simulink model "Torque_Vectoring_Controller_Boon"  (R2016a)
settings: Solver=ode45  StartTime=0.0  StopTime=inf  RelTol=1e-3
InitFcn:
  | clear_close
  | dataCar
  | optParam
  | structSensors
  | structSettings
  | structEstimPar
  | structAero
  | structVariables
  | readFuzzyFile
StartFcn:
  | clear_close
  | dataCar
  | optParam
  | structSensors
  | structSettings
  | structEstimPar
  | structAero
  | structVariables
  | readFuzzyFile
values from neighbouring files (symbols this model uses):
  mu = [0.05;0.05;0.05;0.05]    [frictionfrank.m]
undefined symbols (not defined in the file or in its folder): car, optPar, tire_radius
libraries: CarMaker4SL x42, simulink x11, fuzblock x1
(part 1 of 3)
settings Model: ExtModeAutoUpdateStatusClock=off  Creator=fh  LastModifiedBy=Boon
settings DataIOCC: LimitDataPoints=on  SaveFormat=Array  SignalLoggingSaveFormat=ModelDataLogs  SignalLoggingName=sigsOut
settings OptimizationCC: BooleanDataType=off  ExpressionDepthLimit=2147483647  InitFltsAndDblsToZero=on
settings DebuggingCC: SaveWithParameterizedLinksMsg=none  UnderspecifiedInitializationDetection=Classic  MergeDetectMultiDrivingBlocksExec=none  SignalResolutionControl=TryResolveAllWithWarning  MultiTaskDSMMsg=warning  MultiTaskCondExecSysMsg=none  FcnCallInpInsideContextMsg=EnableAllAsWarning  StateNameClashWarn=warning
settings HardwareCC: ProdBitPerPointer=32  ProdLargestAtomicFloat=None  ProdIntDivRoundTo=Undefined  ProdEndianess=Unspecified  ProdWordSize=32  ProdHWDeviceType=32-bit Generic  TargetUnknown=on
settings ModelReferenceCC: PropagateSignalLabelsOutOfModel=off
settings CodeAppCC: MaxIdLength=63
settings GRTTargetCC: TargetFcnLib=ansi_tfl_tmw.mat  CombineOutputUpdateFcns=off  GRTInterface=on

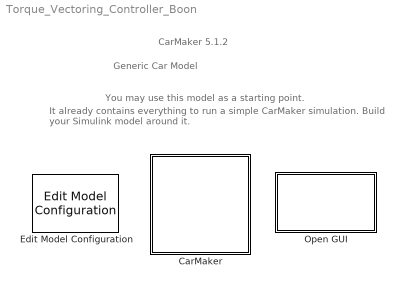
== system Torque_Vectoring_Controller_Boon ==
  note: Generic Car Model
  note: You may use this model as a starting point.
  note: It already contains everything to run a simple CarMaker simulation.
      | Build your Simulink model around it.
  note: CarMaker 5.1.2
  CarMaker : Subsystem  TreatAsAtomicUnit=on
      mask Display: image(imread('CarMaker4SLss.bmp'));
  Edit Model Configuration : CarMaker4SL/Edit Model Configuration
  Open GUI : Subsystem  LoadFcn=if ~length(which('cmcmd')), cmenv; end
      settings: OpenFcn=cmblockmagic('gui_fix_display'); CM_Simulink
      mask Display: image(imread('CarMakerGUI.bmp'));

== system Torque_Vectoring_Controller_Boon/CarMaker ==
  CM_FIRST : Subsystem
  CM_LAST : Subsystem
  Controls : Subsystem
  DrivMan : Subsystem
  Ground : Ground
  IPG Feedback : Subsystem
  IPG Vehicle : Subsystem  TreatAsAtomicUnit=on
  Terminator : Terminator
  Vehicle Sensors : Subsystem
  VehicleControl : Subsystem
  Write CM Dict : CarMaker4SL/Write CM Dict  Commented=on  xname=PT.WFL.Trq_Drive  xsync=off
  Write CM Dict1 : CarMaker4SL/Write CM Dict  Commented=on  xname=PT.WFR.Trq_Drive  xsync=off
  Write CM Dict2 : CarMaker4SL/Write CM Dict  Commented=on  xname=PT.WRL.Trq_Drive  xsync=off
  Write CM Dict3 : CarMaker4SL/Write CM Dict  Commented=on  xname=PT.WRR.Trq_Drive  xsync=off
  wires:
  DrivMan/2(DrivMan.Out) -> VehicleControl/2(DrivMan.In)
  DrivMan/1(Sync_Out) -> VehicleControl/1(Sync_In)
  CM_FIRST/2(Env.Misc) -> DrivMan/2(Env.Misc)
  CM_FIRST/1(Sync_Out) -> DrivMan/1(Sync_In)
  CM_LAST/1(Sync_Out) -> Terminator/1
  IPG Vehicle/1(Sync_Out) -> CM_LAST/1(Sync_In)
  VehicleControl/1(Sync_Out) -> IPG Vehicle/1(Sync_In)
  VehicleControl/3(VhclCtrl.Steering) -> IPG Vehicle/3(VhclCtrl.Steering)
  VehicleControl/4(Vhcl.Wheel.In) -> IPG Vehicle/4(Vhcl.Wheel.In)
  VehicleControl/5(Vhcl.Misc) -> IPG Vehicle/5(Vhcl.Misc)
  VehicleControl/6(VhclCtrl.Brake) -> IPG Vehicle/6(VhclCtrl.Brake)
  VehicleControl/7(VhclCtrl.PT) -> IPG Vehicle/7(VhclCtrl.PT)
  VehicleControl/2(Vhcl.Model.Source) -> IPG Vehicle/2(Vhcl.Model.Source)
  Ground/1 -> CM_FIRST/1(Sync_In)
  Vehicle Sensors/1(" Sensor Bus") -> Controls/1(Sensor Bus)
  Controls/1(Torque Bus) -> IPG Feedback/1(Torques)
  Vehicle Sensors/2(wheelspeeds) -> IPG Feedback/2(Wheelspeeds)

== system Torque_Vectoring_Controller_Boon/Open GUI ==
  S-Function : S-Function  FunctionName=cm_gui  SFunctionDeploymentMode=off  EnableBusSupport=off

== system Torque_Vectoring_Controller_Boon/CarMaker/CM_FIRST ==
  Sync_In : Inport
  Bus Creator1 : BusCreator  Inputs=9
  Demux : Demux  Outputs=9
  Environment : S-Function  FunctionName=CM_Sfun  Parameters='Environment'  SFunctionDeploymentMode=off  EnableBusSupport=off
  IoIn : S-Function  FunctionName=CM_Sfun  Parameters='IoIn'  SFunctionDeploymentMode=off  EnableBusSupport=off
  Sync_Out : Outport
  Env.Misc : Outport  Port=2
  wires:
  Bus Creator1/1 -> Env.Misc/1
  Environment/2 -> Demux/1
  Demux/4 -> Bus Creator1/4  "Env AirHumidity"
  Demux/3 -> Bus Creator1/3  "Env AirPressure"
  Demux/2 -> Bus Creator1/2  "Env AirDensity"
  Demux/1 -> Bus Creator1/1  "Env Temperature"
  Environment/1 -> Sync_Out/1
  IoIn/1 -> Environment/1
  Sync_In/1 -> IoIn/1
  Demux/5 -> Bus Creator1/5  "Env Time"
  Demux/6 -> Bus Creator1/6  "Env SolarRadiation"
  Demux/7 -> Bus Creator1/7  "Env WindVel_tot x"
  Demux/8 -> Bus Creator1/8  "Env WindVel_tot y"
  Demux/9 -> Bus Creator1/9  "Env WindVel_tot z"

== system Torque_Vectoring_Controller_Boon/CarMaker/CM_LAST ==
  Sync_In : Inport
  CM_User : S-Function  FunctionName=CM_Sfun  Parameters='CM_User'  SFunctionDeploymentMode=off  EnableBusSupport=off
  IoOut : S-Function  FunctionName=CM_Sfun  Parameters='IoOut'  SFunctionDeploymentMode=off  EnableBusSupport=off
  Sync_Out : Outport
  wires:
  IoOut/1 -> Sync_Out/1
  CM_User/1 -> IoOut/1
  Sync_In/1 -> CM_User/1

== system Torque_Vectoring_Controller_Boon/CarMaker/Controls ==
  Sensor Bus : Inport
  Control Systems : Subsystem
  Controller Settings : Subsystem
  Vehicle Estimated Parameters : Subsystem
  Torque Bus : Outport
  wires:
  Control Systems/1(Torques) -> Torque Bus/1
  Sensor Bus/1 -> Controller Settings/1(Sensor Bus), Control Systems/1(Sensor Bus), Vehicle Estimated Parameters/1(Sensor Bus)
  [Settings] -> Vehicle Estimated Parameters/2(Settings)
  Vehicle Estimated Parameters/1(" estimParBus") -> Control Systems/4(estimParBus)
  Controller Settings/1(Settings) -> [Settings]
  [Settings] -> Control Systems/2(Settings)
  Controller Settings/2(Variables) -> [Variables]
  [Variables] -> Control Systems/3("Variables ")

== system Torque_Vectoring_Controller_Boon/CarMaker/DrivMan ==
  note: There's rarely a reason to override DrivMan signals.
      | Use the VehicleControl interface for this purpose.
  Sync_In : Inport
  Env.Misc : Inport  Port=2
  BusCreator : BusCreator  Inputs=17
  Demux : Demux  Outputs=17
  DrivMan : S-Function  FunctionName=CM_Sfun  Parameters='DrivMan'  SFunctionDeploymentMode=off  EnableBusSupport=off
  Sync_Out : Outport
  DrivMan.Out : Outport  Port=2
  wires:
  Demux/17 -> BusCreator/17  "DrivMan Steering Trq"
  Demux/16 -> BusCreator/16  "DrivMan Steering AngAcc"
  Demux/15 -> BusCreator/15  "DrivMan Steering AngVel"
  Demux/14 -> BusCreator/14  "DrivMan Steering Ang"
  Demux/13 -> BusCreator/13  "DrivMan Gas"
  Demux/12 -> BusCreator/12  "DrivMan Clutch"
  Demux/11 -> BusCreator/11  "DrivMan BrakePark"
  Demux/10 -> BusCreator/10  "DrivMan Brake"
  Demux/9 -> BusCreator/9  "DrivMan GearNo"
  Demux/8 -> BusCreator/8  "DrivMan SelectorCtrl"
  Demux/7 -> BusCreator/7  "DrivMan UserSignal4"
  Demux/6 -> BusCreator/6  "DrivMan UserSignal3"
  Demux/5 -> BusCreator/5  "DrivMan UserSignal2"
  Demux/4 -> BusCreator/4  "DrivMan UserSignal1"
  Demux/3 -> BusCreator/3  "DrivMan UserSignal0"
  Demux/2 -> BusCreator/2  "DrivMan Key"
  Demux/1 -> BusCreator/1  "DrivMan SST"
  Env.Misc/1 -> DrivMan/2
  Sync_In/1 -> DrivMan/1
  DrivMan/1 -> Sync_Out/1
  BusCreator/1 -> DrivMan.Out/1
  DrivMan/2 -> Demux/1

== system Torque_Vectoring_Controller_Boon/CarMaker/IPG Feedback ==
  Torques : Inport
  Wheelspeeds : Inport  Port=2
  Constant : Constant  Value=1200  VectorParams1D=off  SampleTime=-1
  Demux : Demux
  Subsystem : Subsystem
  wires:
  Demux/3 -> Subsystem/3(Torque_MotRL)
  Torques/1 -> Demux/1
  Constant/1 -> Subsystem/8(WheelspeedLimitRR_RPM), Subsystem/7(WheelspeedLimitRL_RPM), Subsystem/6(WheelspeedLimitFR_RPM), Subsystem/5(WheelspeedLimitFL_RPM)
  Demux/2 -> Subsystem/2(Torque_MotFR)
  Wheelspeeds/1 -> Subsystem/9(SensorBus)
  Demux/1 -> Subsystem/1(Torque_MotFL)
  Demux/4 -> Subsystem/4(Torque_MotRR)

== system Torque_Vectoring_Controller_Boon/CarMaker/IPG Vehicle ==
  Sync_In : Inport
  Vhcl.Model.Source : Inport  Port=2
  VhclCtrl.Steering : Inport  Port=3
  Vhcl.Wheel.In : Inport  Port=4
  Vhcl.Misc : Inport  Port=5
  VhclCtrl.Brake : Inport  Port=6
  VhclCtrl.PT : Inport  Port=7
  Brake : Subsystem
  CarAndTrailer : Subsystem
  PowerTrain : Subsystem
  Stop Simulation : Stop
  VehicleSource_BuiltIn : simulink/Logic and Bit Operations/Compare To Constant  relop=~=  const=1  OutDataTypeStr=boolean  ZeroCross=off
  Sync_Out : Outport
  wires:
  VhclCtrl.PT/1 -> PowerTrain/3(VhclCtrl.PT)
  Brake/1(Sync_Out) -> PowerTrain/1(Sync_In)
  CarAndTrailer/1(Sync_Out) -> Brake/1(Sync_In)
  CarAndTrailer/2(Brake.IF.In) -> Brake/2(Brake.IF.In)
  VhclCtrl.Brake/1 -> Brake/3(VhclCtrl.Brake)
  PowerTrain/1(Sync_Out) -> Sync_Out/1
  Vhcl.Misc/1 -> CarAndTrailer/4(Vhcl.Misc)
  Vhcl.Wheel.In/1 -> CarAndTrailer/3(Vhcl.Wheel.In)
  VhclCtrl.Steering/1 -> CarAndTrailer/2(VhclCtrl.Steering)
  Sync_In/1 -> CarAndTrailer/1(Sync_In)
  Vhcl.Model.Source/1 -> VehicleSource_BuiltIn/1
  VehicleSource_BuiltIn/1 -> Stop Simulation/1
  Brake/2(Vhcl.Wheel.PT) -> PowerTrain/2(Vhcl.Wheel.PT)

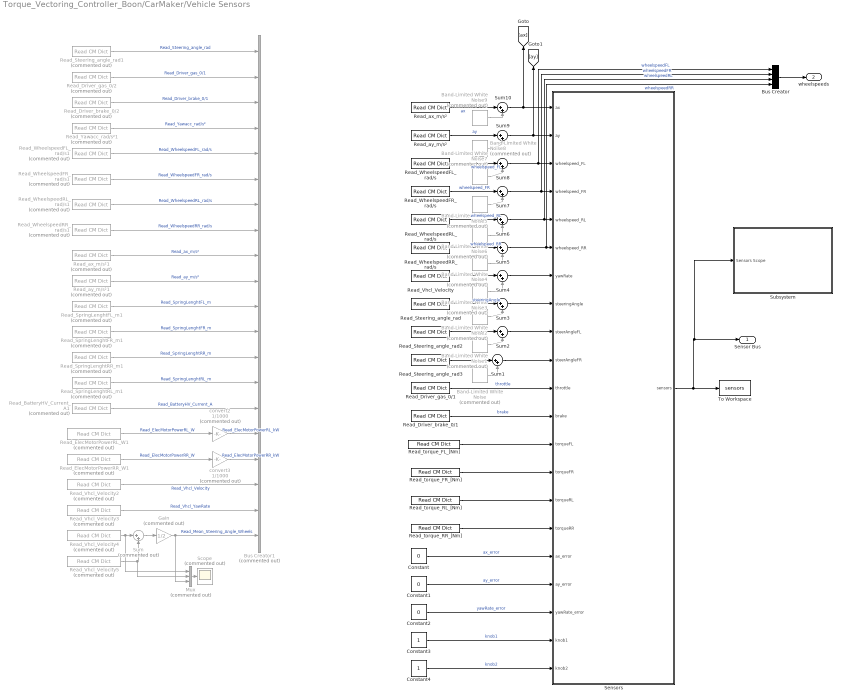
== system Torque_Vectoring_Controller_Boon/CarMaker/Vehicle Sensors ==
  Band-Limited White Noise{,1..9} (10 alike) : simulink/Sources/Band-Limited White Noise  Commented=on  Cov=[0.00000001]  Ts=car.dt  seed=[23341]
  Bus Creator : BusCreator  Inputs=4
  Bus Creator1 : BusCreator  Commented=on  Inputs=20
  Constant : Constant  Value=0
  Constant1 : Constant  Value=0
  Constant2 : Constant  Value=0
  Constant3 : Constant
  Constant4 : Constant
  Gain : Gain  Commented=on  Gain=1/2
  Mux : Mux  Commented=on  Inputs=3
  Read_BatteryHV_Current_A1 : CarMaker4SL/Read CM Dict  Commented=on  xname=PT.BattHV.Current  xsync=off
  Read_Driver_brake_0/1 : CarMaker4SL/Read CM Dict  xname=DM.Brake  xsync=off
  Read_Driver_brake_0/2 : CarMaker4SL/Read CM Dict  Commented=on  xname=DM.Brake  xsync=off
  Read_Driver_gas_0/1 : CarMaker4SL/Read CM Dict  xname=DM.Gas  xsync=off
  Read_Driver_gas_0/2 : CarMaker4SL/Read CM Dict  Commented=on  xname=DM.Gas  xsync=off
  Read_ElecMotorPowerRL_W1 : CarMaker4SL/Read CM Dict  Commented=on  xname=PT.Motor.PwrElec  xsync=off
  Read_ElecMotorPowerRR_W1 : CarMaker4SL/Read CM Dict  Commented=on  xname=PT.Motor1.PwrElec  xsync=off
  Read_SpringLenghtFL_m1 : CarMaker4SL/Read CM Dict  Commented=on  xname=Car.SpringFL.l  xsync=off
  Read_SpringLenghtFR_m1 : CarMaker4SL/Read CM Dict  Commented=on  xname=Car.SpringFR.l  xsync=off
  Read_SpringLenghtRL_m1 : CarMaker4SL/Read CM Dict  Commented=on  xname=Car.SpringRL.l  xsync=off
  Read_SpringLenghtRR_m1 : CarMaker4SL/Read CM Dict  Commented=on  xname=Car.SpringRR.l  xsync=off
  Read_Steering_angle_rad : CarMaker4SL/Read CM Dict  xname=Steer.WhlAng  xsync=off
  Read_Steering_angle_rad1 : CarMaker4SL/Read CM Dict  Commented=on  xname=Steer.WhlAng  xsync=off
  Read_Steering_angle_rad2 : CarMaker4SL/Read CM Dict  xname=Car.SteerAngleFL  xsync=off
  Read_Steering_angle_rad3 : CarMaker4SL/Read CM Dict  xname=Car.SteerAngleFR  xsync=off
  Read_Vhcl_Velocity : CarMaker4SL/Read CM Dict  xname=Vhcl.YawRate  xsync=off
  Read_Vhcl_Velocity2 : CarMaker4SL/Read CM Dict  Commented=on  xname=Vhcl.v  xsync=off
  Read_Vhcl_Velocity3 : CarMaker4SL/Read CM Dict  Commented=on  xname=Vhcl.YawRate  xsync=off
  Read_Vhcl_Velocity4 : CarMaker4SL/Read CM Dict  Commented=on  xname=Car.SteerAngleFL  xsync=off
  Read_Vhcl_Velocity5 : CarMaker4SL/Read CM Dict  Commented=on  xname=Car.SteerAngleFR  xsync=off
  Read_WheelspeedFL_rad/s : CarMaker4SL/Read CM Dict  xname=Vhcl.FL.rotv  xsync=off
  Read_WheelspeedFL_rad/s1 : CarMaker4SL/Read CM Dict  Commented=on  xname=Vhcl.FL.rotv  xsync=off
  Read_WheelspeedFR_rad/s : CarMaker4SL/Read CM Dict  xname=Vhcl.FR.rotv  xsync=off
  Read_WheelspeedFR_rad/s1 : CarMaker4SL/Read CM Dict  Commented=on  xname=Vhcl.FR.rotv  xsync=off
  Read_WheelspeedRL_rad/s : CarMaker4SL/Read CM Dict  xname=Vhcl.RL.rotv  xsync=off
  Read_WheelspeedRL_rad/s1 : CarMaker4SL/Read CM Dict  Commented=on  xname=Vhcl.RL.rotv  xsync=off
  Read_WheelspeedRR_rad/s : CarMaker4SL/Read CM Dict  xname=Vhcl.RR.rotv  xsync=off
  Read_WheelspeedRR_rad/s1 : CarMaker4SL/Read CM Dict  Commented=on  xname=Vhcl.RR.rotv  xsync=off
  Read_Yawacc_rad/s²1 : CarMaker4SL/Read CM Dict  Commented=on  xname=Vhcl.YawAcc  xsync=off
  Read_ax_m/s² : CarMaker4SL/Read CM Dict  xname=Car.ax  xsync=off
  Read_ax_m/s²1 : CarMaker4SL/Read CM Dict  Commented=on  xname=Car.ax  xsync=off
  Read_ay_m/s² : CarMaker4SL/Read CM Dict  xname=Car.ay  xsync=off
  Read_ay_m/s²1 : CarMaker4SL/Read CM Dict  Commented=on  xname=Car.ay  xsync=off
  Read_torque_FL_[Nm] : CarMaker4SL/Read CM Dict  xname=PT.WFL.Trq_Drive  xsync=off
  Read_torque_FR_[Nm] : CarMaker4SL/Read CM Dict  xname=PT.WFR.Trq_Drive  xsync=off
  Read_torque_RL_[Nm] : CarMaker4SL/Read CM Dict  xname=PT.WRL.Trq_Drive  xsync=off
  Read_torque_RR_[Nm] : CarMaker4SL/Read CM Dict  xname=PT.WRR.Trq_Drive  xsync=off
  Scope : Scope  Commented=on
  Sensors : MATLAB Function  TreatAsAtomicUnit=on
  Subsystem : Subsystem
      mask Display: image('Sensors Scope.png');
  Sum : Sum  Commented=on  Inputs=|++
  Sum{1..10} (10 alike) : Sum  Inputs=|++
  To Workspace : ToWorkspace  VariableName=sensors  SaveFormat=Timeseries  SampleTime=-1
  convert2 : Gain  Commented=on  Gain=1/1000
  convert3 : Gain  Commented=on  Gain=1/1000
  " Sensor Bus" : Outport
  wheelspeeds : Outport  Port=2
  wires:
  Mux/1 -> Scope/1
  Gain/1 -> Bus Creator1/20, Mux/3  "Read_Mean_Steering_Angle_Wheels"
  Sum/1 -> Gain/1
  Read_Vhcl_Velocity5/1 -> Sum/2, Mux/2
  Read_Vhcl_Velocity4/1 -> Sum/1, Mux/1
  Read_Vhcl_Velocity3/1 -> Bus Creator1/19  "Read_Vhcl_YawRate"
  Read_Vhcl_Velocity2/1 -> Bus Creator1/18  "Read_Vhcl_Velocity"
  convert3/1 -> Bus Creator1/17  "Read_ElecMotorPowerRR_kW"
  convert2/1 -> Bus Creator1/16  "Read_ElecMotorPowerRL_kW"
  Read_ElecMotorPowerRR_W1/1 -> convert3/1  "Read_ElecMotorPowerRR_W"
  Read_ElecMotorPowerRL_W1/1 -> convert2/1  "Read_ElecMotorPowerRL_W"
  Read_BatteryHV_Current_A1/1 -> Bus Creator1/15  "Read_BatteryHV_Current_A"
  Read_SpringLenghtRR_m1/1 -> Bus Creator1/13  "Read_SpringLenghtRR_m"
  Read_SpringLenghtRL_m1/1 -> Bus Creator1/14  "Read_SpringLenghtRL_m"
  Read_SpringLenghtFR_m1/1 -> Bus Creator1/12  "Read_SpringLenghtFR_m"
  Read_SpringLenghtFL_m1/1 -> Bus Creator1/11  "Read_SpringLenghtFL_m"
  Read_ay_m/s²1/1 -> Bus Creator1/10  "Read_ay_m/s²"
  Read_ax_m/s²1/1 -> Bus Creator1/9  "Read_ax_m/s²"
  Read_WheelspeedRR_rad/s1/1 -> Bus Creator1/8  "Read_WheelspeedRR_rad/s"
  Read_WheelspeedRL_rad/s1/1 -> Bus Creator1/7  "Read_WheelspeedRL_rad/s"
  Read_WheelspeedFR_rad/s1/1 -> Bus Creator1/6  "Read_WheelspeedFR_rad/s"
  Read_WheelspeedFL_rad/s1/1 -> Bus Creator1/5  "Read_WheelspeedFL_rad/s"
  Read_Yawacc_rad/s²1/1 -> Bus Creator1/4  "Read_Yawacc_rad/s²"
  Read_Driver_brake_0/2/1 -> Bus Creator1/3  "Read_Driver_brake_0/1"
  Read_Driver_gas_0/2/1 -> Bus Creator1/2  "Read_Driver_gas_0/1"
  Read_Steering_angle_rad1/1 -> Bus Creator1/1  "Read_Steering_angle_rad"
  Constant4/1 -> Sensors/21(knob2)  "knob2"
  Constant3/1 -> Sensors/20(knob1)  "knob1"
  Constant2/1 -> Sensors/19(yawRate_error)  "yawRate_error"
  Constant1/1 -> Sensors/18(ay_error)  "ay_error"
  Constant/1 -> Sensors/17(ax_error)  "ax_error"
  Sensors/1(sensors) -> Subsystem/1("Sensors Scope "), " Sensor Bus"/1, To Workspace/1
  Read_Driver_brake_0/1/1 -> Sensors/12(brake)  "brake"
  Read_Driver_gas_0/1/1 -> Sensors/11(throttle)  "throttle"
  Bus Creator/1 -> wheelspeeds/1
  Read_torque_FL_[Nm]/1 -> Sensors/13(torqueFL)
  Read_torque_RR_[Nm]/1 -> Sensors/16(torqueRR)
  Read_torque_RL_[Nm]/1 -> Sensors/15(torqueRL)
  Read_torque_FR_[Nm]/1 -> Sensors/14(torqueFR)
  Read_Steering_angle_rad3/1 -> Sum1/1
  Sum1/1 -> Sensors/10(steerAngleFR)
  Band-Limited White Noise/1 -> Sum1/2
  Sum2/1 -> Sensors/9(steerAngleFL)
  Read_Steering_angle_rad2/1 -> Sum2/1
  Band-Limited White Noise1/1 -> Sum2/2
  Sum3/1 -> Sensors/8(steeringAngle)
  Read_Steering_angle_rad/1 -> Sum3/1  "steeringAngle"
  Band-Limited White Noise2/1 -> Sum3/2
  Sum4/1 -> Sensors/7(yawRate)
  Read_Vhcl_Velocity/1 -> Sum4/1
  Band-Limited White Noise3/1 -> Sum4/2
  Sum5/1 -> Bus Creator/4, Sensors/6(wheelspeed_RR)  "wheelspeedRR"
  Read_WheelspeedRR_rad/s/1 -> Sum5/1  "wheelspeed_RR"
  Band-Limited White Noise4/1 -> Sum5/2
  Sum6/1 -> Bus Creator/3, Sensors/5(wheelspeed_RL)  "wheelspeedRL"
  Read_WheelspeedRL_rad/s/1 -> Sum6/1  "wheelspeed_RL"
  Band-Limited White Noise6/1 -> Sum6/2
  Band-Limited White Noise5/1 -> Sum7/2
  Read_WheelspeedFR_rad/s/1 -> Sum7/1  "wheelspeed_FR"
  Sum7/1 -> Bus Creator/2, Sensors/4(wheelspeed_FR)  "wheelspeedFR"
  Read_WheelspeedFL_rad/s/1 -> Sum8/1  "wheelspeed_FL"
  Sum8/1 -> Bus Creator/1, Sensors/3(wheelspeed_FL)  "wheelspeedFL"
  Band-Limited White Noise7/1 -> Sum8/2
  Band-Limited White Noise8/1 -> Sum9/2
  Read_ay_m/s²/1 -> Sum9/1  "ay"
  Sum9/1 -> Sensors/2(ay), [ay]
  Band-Limited White Noise9/1 -> Sum10/2
  Read_ax_m/s²/1 -> Sum10/1  "ax"
  Sum10/1 -> Sensors/1(ax), [ax]

== system Torque_Vectoring_Controller_Boon/CarMaker/VehicleControl ==
  note: <Your model here>
  note: When implementing a vehicle control model,
      | be sure to add '-disablevehiclecontrol' to the command line arguments
      | in the CarMaker Model Configuration block.
      | Otherwise your model will possibly not see the original DrivMan signals
      | on its inputs, but those of a currently activated C-coded vehicle control model instead.
  Sync_In : Inport
  DrivMan.In : Inport  Port=2
  Bus Creator2 : BusCreator  Inputs=2
  CreateBus Vhcl.Misc : Subsystem
  CreateBus Vhcl.Wheel.In : Subsystem
  CreateBus VhclCtrl : Subsystem
  CreateBus VhclCtrl.PT : Subsystem
  CreateBus VhclCtrl.Steering : Subsystem
  Demux2 : Demux  Outputs=2
  VehicleControl : S-Function  FunctionName=CM_Sfun  Parameters='VehicleControl'  SFunctionDeploymentMode=off  EnableBusSupport=off
  VehicleControlUpd : S-Function  FunctionName=CM_Sfun  Parameters='VehicleControlUpd'  SFunctionDeploymentMode=off  EnableBusSupport=off
  Sync_Out : Outport
  Vhcl.Model.Source : Outport  Port=2
  VhclCtrl.Steering : Outport  Port=3
  Vhcl.Wheel.In : Outport  Port=4
  Vhcl.Misc : Outport  Port=5
  VhclCtrl.Brake : Outport  Port=6
  VhclCtrl.PT : Outport  Port=7
  wires:
  CreateBus VhclCtrl/1(Out) -> VehicleControlUpd/2
  VehicleControl/2 -> CreateBus VhclCtrl/1(In)
  VehicleControlUpd/2 -> Vhcl.Model.Source/1
  VehicleControlUpd/4 -> CreateBus Vhcl.Wheel.In/1(In1)
  VehicleControlUpd/5 -> CreateBus Vhcl.Misc/1(In1)
  VehicleControlUpd/6 -> Demux2/1
  VehicleControlUpd/7 -> CreateBus VhclCtrl.PT/1(In1)
  VehicleControlUpd/3 -> CreateBus VhclCtrl.Steering/1(In1)
  CreateBus Vhcl.Misc/1(Out1) -> Vhcl.Misc/1
  CreateBus Vhcl.Wheel.In/1(Out1) -> Vhcl.Wheel.In/1
  DrivMan.In/1 -> VehicleControl/2
  VehicleControl/1 -> VehicleControlUpd/1
  Sync_In/1 -> VehicleControl/1
  CreateBus VhclCtrl.PT/1(Out1) -> VhclCtrl.PT/1
  Bus Creator2/1 -> VhclCtrl.Brake/1
  CreateBus VhclCtrl.Steering/1(Out1) -> VhclCtrl.Steering/1
  VehicleControlUpd/1 -> Sync_Out/1
  Demux2/2 -> Bus Creator2/2  "VhclCtrl BrakePark"
  Demux2/1 -> Bus Creator2/1  "VhclCtrl Brake"

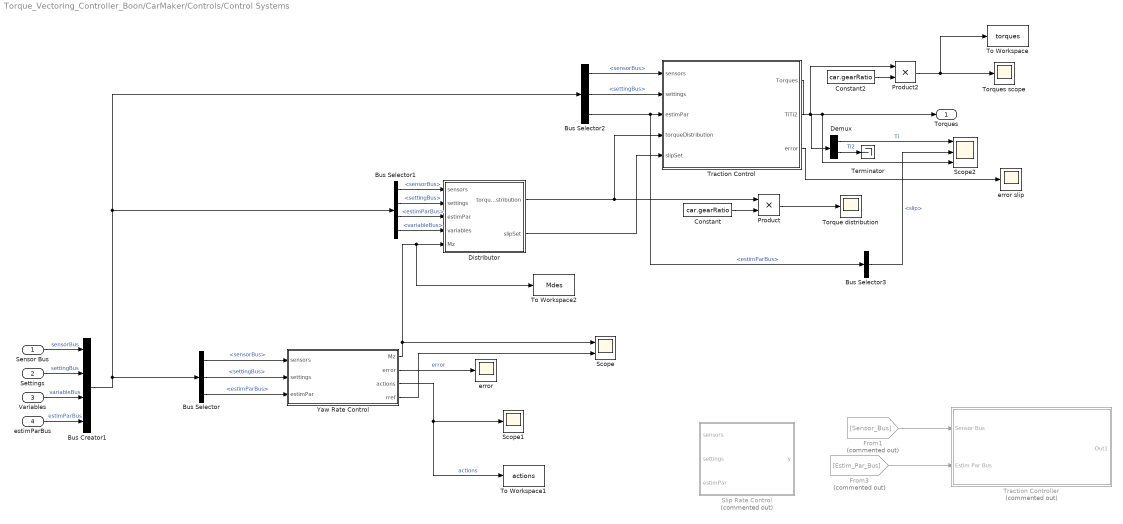
== system Torque_Vectoring_Controller_Boon/CarMaker/Controls/Control Systems ==
  Sensor Bus : Inport
  Settings : Inport  Port=2
  "Variables " : Inport  Port=3
  estimParBus : Inport  Port=4
  Bus Creator1 : BusCreator  Inputs=4
  Bus Selector : BusSelector  OutputSignals=sensorBus,settingBus,estimParBus
  Bus Selector1 : BusSelector  OutputSignals=sensorBus,settingBus,estimParBus,variableBus
  Bus Selector2 : BusSelector  OutputSignals=sensorBus,settingBus,estimParBus
  Bus Selector3 : BusSelector  OutputSignals=slip
  Constant : Constant  Value=car.gearRatio
  Constant2 : Constant  Value=car.gearRatio
  Demux : Demux  Outputs=2
  Distributor : Subsystem
  From1 : From  Commented=on  GotoTag=Sensor_Bus  TagVisibility=global
  From3 : From  Commented=on  GotoTag=Estim_Par_Bus  TagVisibility=global
  Product : Product
  Product2 : Product
  Scope : Scope  NumInputPorts=2
  Scope1 : Scope
  Scope2 : Scope  NumInputPorts=3
  Slip Rate Control : MATLAB Function  Commented=on  TreatAsAtomicUnit=on
  Terminator : Terminator
  To Workspace : ToWorkspace  VariableName=torques  SaveFormat=Timeseries  SampleTime=-1
  To Workspace1 : ToWorkspace  VariableName=actions  SaveFormat=Timeseries  SampleTime=-1
  To Workspace2 : ToWorkspace  VariableName=Mdes  SaveFormat=Timeseries  SampleTime=-1
  Torque distribution : Scope
  Torques scope : Scope
  Traction Control : MATLAB Function  TreatAsAtomicUnit=on
  Traction Controller : Subsystem  Commented=on
  Yaw Rate Control : MATLAB Function  TreatAsAtomicUnit=on
  error : Scope
  error slip : Scope
  Torques : Outport
  wires:
  From1/1 -> Traction Controller/1(Sensor Bus)
  From3/1 -> Traction Controller/2(Estim Par Bus)
  Yaw Rate Control/1(Mz) -> To Workspace2/1, Distributor/5(Mz), Scope/1
  Settings/1 -> Bus Creator1/2  "settingBus"
  Sensor Bus/1 -> Bus Creator1/1  "sensorBus"
  Bus Selector/2 -> Yaw Rate Control/2(settings)  "<settingBus>"
  Bus Selector/1 -> Yaw Rate Control/1(sensors)  "<sensorBus>"
  Bus Selector1/3 -> Distributor/3(estimPar)  "<estimParBus>"
  Bus Selector1/2 -> Distributor/2(settings)  "<settingBus>"
  Bus Selector1/1 -> Distributor/1(sensors)  "<sensorBus>"
  Distributor/1(torqueDistribution) -> Product/1, Traction Control/4(torqueDistribution)
  Bus Selector2/3 -> Bus Selector3/1, Traction Control/3(estimPar)  "<estimParBus>"
  Bus Selector2/2 -> Traction Control/2(settings)  "<settingBus>"
  Bus Selector2/1 -> Traction Control/1(sensors)  "<sensorBus>"
  Bus Creator1/1 -> Bus Selector2/1, Bus Selector1/1, Bus Selector/1
  Bus Selector/3 -> Yaw Rate Control/3(estimPar)  "<estimParBus>"
  Distributor/2(slipSet) -> Traction Control/5(slipSet)
  Yaw Rate Control/2(error) -> error/1  "error"
  Yaw Rate Control/3(actions) -> To Workspace1/1, Scope1/1  "actions"
  estimParBus/1 -> Bus Creator1/4  "estimParBus"
  "Variables "/1 -> Bus Creator1/3  "variableBus"
  Bus Selector1/4 -> Distributor/4(variables)  "<variableBus>"
  Yaw Rate Control/4(rref) -> Scope/2
  Product/1 -> Torque distribution/1
  Constant/1 -> Product/2
  Traction Control/1(Torques) -> Product2/1, Torques/1, Scope2/3
  Constant2/1 -> Product2/2
  Product2/1 -> To Workspace/1, Torques scope/1
  Traction Control/2(TiTi2) -> Demux/1
  Demux/1 -> Scope2/1  "Ti"
  Traction Control/3(error) -> error slip/1
  Demux/2 -> Terminator/1  "Ti2"
  Bus Selector3/1 -> Scope2/2  "<slip>"

== system Torque_Vectoring_Controller_Boon/CarMaker/Controls/Controller Settings ==
  Sensor Bus : Inport
  Controller Settings : MATLAB Function  TreatAsAtomicUnit=on
  To Workspace : ToWorkspace  VariableName=settingOut  SaveFormat=Timeseries  SampleTime=-1
  Settings : Outport
  Variables : Outport  Port=2
  wires:
  Sensor Bus/1 -> Controller Settings/1(sensors)
  Controller Settings/2(variables) -> Variables/1
  Controller Settings/1(settings) -> To Workspace/1, Settings/1

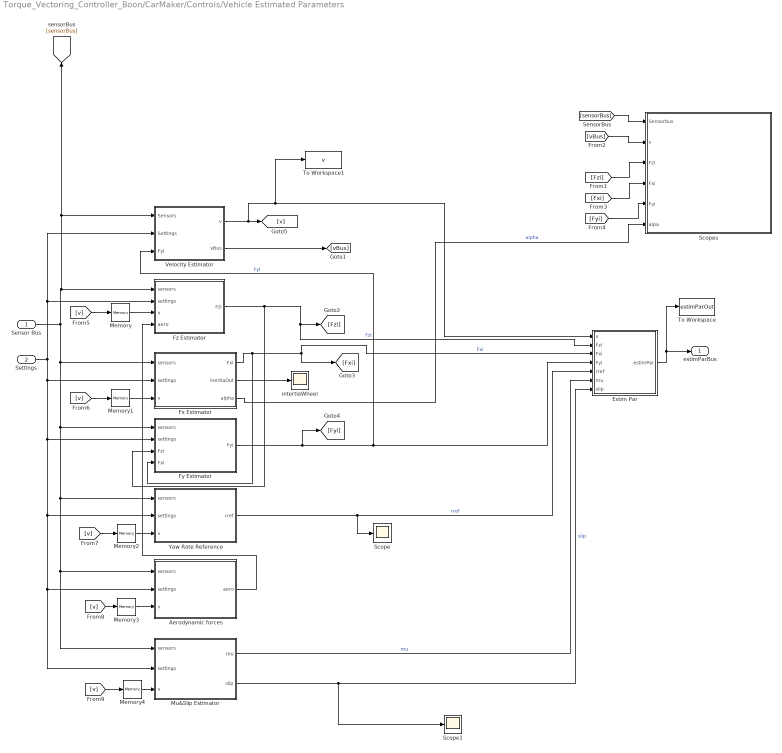
== system Torque_Vectoring_Controller_Boon/CarMaker/Controls/Vehicle Estimated Parameters ==
  Sensor Bus : Inport
  Settings : Inport  Port=2
  Aerodynamic forces : MATLAB Function  TreatAsAtomicUnit=on
  Estim Par : MATLAB Function  TreatAsAtomicUnit=on
  "Fx Estimator " : MATLAB Function  TreatAsAtomicUnit=on
  "Fy Estimator " : MATLAB Function  TreatAsAtomicUnit=on
  "Fz Estimator " : MATLAB Function  TreatAsAtomicUnit=on
  Memory{,1..4} (5 alike) : Memory
  Mu&Slip Estimator : MATLAB Function  TreatAsAtomicUnit=on
  Scope : Scope
  Scope1 : Scope
  Scopes : Subsystem
      mask Display: image('estimator.png');
  To Workspace : ToWorkspace  VariableName=estimParOut  SaveFormat=Timeseries  SampleTime=-1
  To Workspace1 : ToWorkspace  VariableName=v  SaveFormat=Timeseries  SampleTime=-1
  Velocity Estimator : Subsystem
  Yaw Rate Reference : MATLAB Function  TreatAsAtomicUnit=on
  intertiaWheel : Scope
  " estimParBus" : Outport
  wires:
  "Fx Estimator "/1(Fxi) -> Estim Par/3(Fxi), [Fxi], "Fy Estimator "/4(Fxi)  "Fxi"
  "Fz Estimator "/1(Fzi) -> "Fy Estimator "/3(Fzi), [Fzi], Estim Par/2(Fzi)  "Fzi"
  Yaw Rate Reference/1(rref) -> Estim Par/5(rref), Scope/1  "rref"
  "Fy Estimator "/1(Fyi) -> [Fyi], Velocity Estimator/3(Fyi), Estim Par/4(Fyi)  "Fyi"
  Estim Par/1(estimPar) -> To Workspace/1, " estimParBus"/1
  [vBus] -> Scopes/2(v)
  [Fzi] -> Scopes/3(Fzi)
  [sensorBus] -> Scopes/1(Sensorbus)
  [Fxi] -> Scopes/4(Fxi)
  Sensor Bus/1 -> "Fx Estimator "/1(sensors), Mu&Slip Estimator/1(sensors), Aerodynamic forces/1(sensors), Yaw Rate Reference/1(sensors), "Fy Estimator "/1(sensors), "Fz Estimator "/1(sensors), Velocity Estimator/1(Sensors), [sensorBus]
  Settings/1 -> Velocity Estimator/2(Settings), "Fz Estimator "/2(settings), Mu&Slip Estimator/2(settings), Aerodynamic forces/2(settings), Yaw Rate Reference/2(settings), "Fy Estimator "/2(settings), "Fx Estimator "/2(settings)
  [Fyi] -> Scopes/5(Fyi)
  Velocity Estimator/1(v) -> Estim Par/1(v), To Workspace1/1, [v]
  Velocity Estimator/2(vBus) -> [vBus]
  Aerodynamic forces/1(aero) -> "Fz Estimator "/4(aero)
  Mu&Slip Estimator/1(mu) -> Estim Par/6(mu)  "mu"
  Mu&Slip Estimator/2(slip) -> Scope1/1, Estim Par/7(slip)  "slip"
  [v] -> Memory/1
  [v] -> Memory1/1
  [v] -> Memory2/1
  [v] -> Memory3/1
  [v] -> Memory4/1
  "Fx Estimator "/2(inertiaOut) -> intertiaWheel/1
  "Fx Estimator "/3(alpha) -> Scopes/6(alpa)  "alpha"
  Memory/1 -> "Fz Estimator "/3(v)
  Memory1/1 -> "Fx Estimator "/3(v)
  Memory2/1 -> Yaw Rate Reference/3(v)
  Memory3/1 -> Aerodynamic forces/3(v)
  Memory4/1 -> Mu&Slip Estimator/3(v)

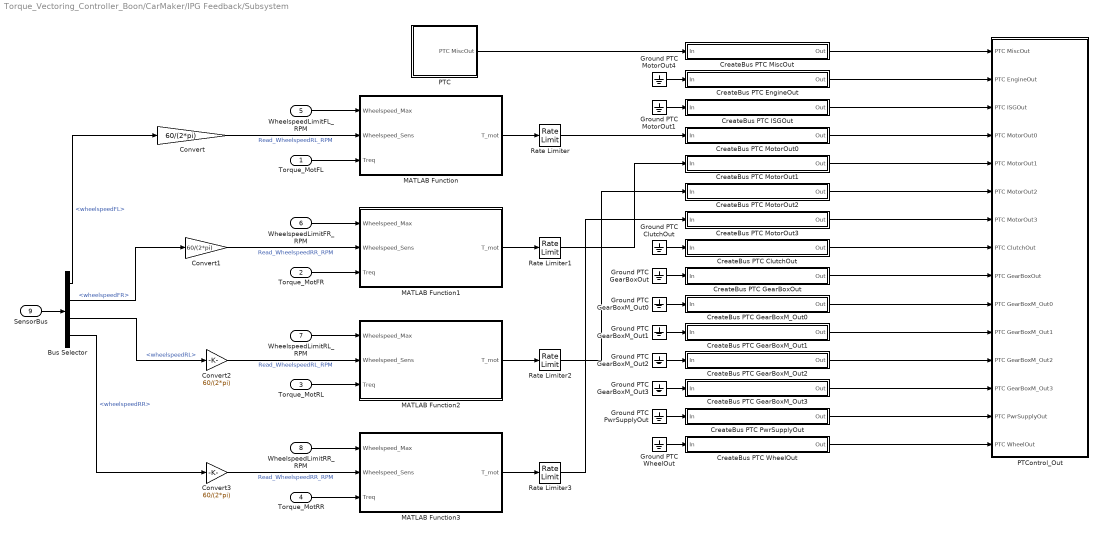
== system Torque_Vectoring_Controller_Boon/CarMaker/IPG Feedback/Subsystem ==
  Torque_MotFL : Inport
  Torque_MotFR : Inport  Port=2
  Torque_MotRL : Inport  Port=3
  Torque_MotRR : Inport  Port=4
  WheelspeedLimitFL_RPM : Inport  Port=5
  WheelspeedLimitFR_RPM : Inport  Port=6
  WheelspeedLimitRL_RPM : Inport  Port=7
  WheelspeedLimitRR_RPM : Inport  Port=8
  SensorBus : Inport  Port=9
  Bus Selector : BusSelector  OutputSignals=wheelspeedFL,wheelspeedFR,wheelspeedRL,wheelspeedRR
  Convert{,1..3} (4 alike) : Gain  Gain=60/(2*pi)
  CreateBus PTC ClutchOut : Subsystem
  CreateBus PTC EngineOut : Subsystem
  CreateBus PTC GearBoxM_Out0 : Subsystem
  CreateBus PTC GearBoxM_Out1 : Subsystem
  CreateBus PTC GearBoxM_Out2 : Subsystem
  CreateBus PTC GearBoxM_Out3 : Subsystem
  CreateBus PTC GearBoxOut : Subsystem
  CreateBus PTC ISGOut : Subsystem
  CreateBus PTC MiscOut : Subsystem
  CreateBus PTC MotorOut0 : Subsystem
  CreateBus PTC MotorOut1 : Subsystem
  CreateBus PTC MotorOut2 : Subsystem
  CreateBus PTC MotorOut3 : Subsystem
  CreateBus PTC PwrSupplyOut : Subsystem
  CreateBus PTC WheelOut : Subsystem
  Ground PTC ClutchOut : Ground
  Ground PTC GearBoxM_Out{0..3} (4 alike) : Ground
  Ground PTC GearBoxOut : Ground
  Ground PTC MotorOut1 : Ground
  Ground PTC MotorOut4 : Ground
  Ground PTC PwrSupplyOut : Ground
  Ground PTC WheelOut : Ground
  MATLAB Function : MATLAB Function  TreatAsAtomicUnit=on
  MATLAB Function1 : MATLAB Function  TreatAsAtomicUnit=on
  MATLAB Function2 : MATLAB Function  TreatAsAtomicUnit=on
  MATLAB Function3 : MATLAB Function  TreatAsAtomicUnit=on
  PTC : Subsystem
  PTControl_Out : Subsystem
  Rate Limiter{,1..3} (4 alike) : RateLimiter  RisingSlewLimit=80  FallingSlewLimit=-80
  wires:
  Ground PTC GearBoxM_Out1/1 -> CreateBus PTC GearBoxM_Out1/1(In)
  CreateBus PTC MotorOut2/1(Out) -> PTControl_Out/6(PTC MotorOut2)
  Ground PTC GearBoxOut/1 -> CreateBus PTC GearBoxOut/1(In)
  CreateBus PTC GearBoxM_Out0/1(Out) -> PTControl_Out/10(PTC GearBoxM_Out0)
  Ground PTC GearBoxM_Out0/1 -> CreateBus PTC GearBoxM_Out0/1(In)
  Ground PTC ClutchOut/1 -> CreateBus PTC ClutchOut/1(In)
  Ground PTC MotorOut4/1 -> CreateBus PTC EngineOut/1(In)
  CreateBus PTC GearBoxM_Out3/1(Out) -> PTControl_Out/13(PTC GearBoxM_Out3)
  CreateBus PTC GearBoxM_Out1/1(Out) -> PTControl_Out/11(PTC GearBoxM_Out1)
  Ground PTC GearBoxM_Out3/1 -> CreateBus PTC GearBoxM_Out3/1(In)
  Ground PTC MotorOut1/1 -> CreateBus PTC ISGOut/1(In)
  Ground PTC PwrSupplyOut/1 -> CreateBus PTC PwrSupplyOut/1(In)
  CreateBus PTC PwrSupplyOut/1(Out) -> PTControl_Out/14(PTC PwrSupplyOut)
  Ground PTC WheelOut/1 -> CreateBus PTC WheelOut/1(In)
  CreateBus PTC WheelOut/1(Out) -> PTControl_Out/15(PTC WheelOut)
  CreateBus PTC MotorOut3/1(Out) -> PTControl_Out/7(PTC MotorOut3)
  CreateBus PTC ISGOut/1(Out) -> PTControl_Out/3(PTC ISGOut)
  CreateBus PTC MotorOut1/1(Out) -> PTControl_Out/5(PTC MotorOut1)
  CreateBus PTC GearBoxM_Out2/1(Out) -> PTControl_Out/12(PTC GearBoxM_Out2)
  CreateBus PTC ClutchOut/1(Out) -> PTControl_Out/8(PTC ClutchOut)
  Ground PTC GearBoxM_Out2/1 -> CreateBus PTC GearBoxM_Out2/1(In)
  CreateBus PTC GearBoxOut/1(Out) -> PTControl_Out/9(PTC GearBoxOut)
  CreateBus PTC EngineOut/1(Out) -> PTControl_Out/2(PTC EngineOut)
  CreateBus PTC MotorOut0/1(Out) -> PTControl_Out/4(PTC MotorOut0)
  CreateBus PTC MiscOut/1(Out) -> PTControl_Out/1(PTC MiscOut)
  PTC/1(PTC MiscOut) -> CreateBus PTC MiscOut/1(In)
  Torque_MotFR/1 -> MATLAB Function1/3(Treq)
  Torque_MotFL/1 -> MATLAB Function/3(Treq)
  MATLAB Function/1(T_mot) -> Rate Limiter/1
  MATLAB Function1/1(T_mot) -> Rate Limiter1/1
  WheelspeedLimitFL_RPM/1 -> MATLAB Function/1(Wheelspeed_Max)
  WheelspeedLimitFR_RPM/1 -> MATLAB Function1/1(Wheelspeed_Max)
  SensorBus/1 -> Bus Selector/1
  Bus Selector/1 -> Convert/1  "<wheelspeedFL>"
  Convert/1 -> MATLAB Function/2(Wheelspeed_Sens)  "Read_WheelspeedRL_RPM"
  Bus Selector/2 -> Convert1/1  "<wheelspeedFR>"
  Convert1/1 -> MATLAB Function1/2(Wheelspeed_Sens)  "Read_WheelspeedRR_RPM"
  Rate Limiter/1 -> CreateBus PTC MotorOut0/1(In)
  Rate Limiter1/1 -> CreateBus PTC MotorOut1/1(In)
  Torque_MotRR/1 -> MATLAB Function3/3(Treq)
  Torque_MotRL/1 -> MATLAB Function2/3(Treq)
  MATLAB Function2/1(T_mot) -> Rate Limiter2/1
  MATLAB Function3/1(T_mot) -> Rate Limiter3/1
  WheelspeedLimitRL_RPM/1 -> MATLAB Function2/1(Wheelspeed_Max)
  WheelspeedLimitRR_RPM/1 -> MATLAB Function3/1(Wheelspeed_Max)
  Bus Selector/3 -> Convert2/1  "<wheelspeedRL>"
  Convert2/1 -> MATLAB Function2/2(Wheelspeed_Sens)  "Read_WheelspeedRL_RPM"
  Bus Selector/4 -> Convert3/1  "<wheelspeedRR>"
  Convert3/1 -> MATLAB Function3/2(Wheelspeed_Sens)  "Read_WheelspeedRR_RPM"
  Rate Limiter2/1 -> CreateBus PTC MotorOut2/1(In)
  Rate Limiter3/1 -> CreateBus PTC MotorOut3/1(In)

== system Torque_Vectoring_Controller_Boon/CarMaker/IPG Vehicle/Brake ==
  note: <Your model here>
  note: When replacing the entire braking system,
      | be sure to add '-disablebrake' to the command line arguments
      | in the CarMaker Model Configuration block.
  Sync_In : Inport
  Brake.IF.In : Inport  Port=2
  VhclCtrl.Brake : Inport  Port=3
  Brake : S-Function  FunctionName=CM_Sfun  Parameters='Brake'  SFunctionDeploymentMode=off  EnableBusSupport=off
  BrakeUpd : S-Function  FunctionName=CM_Sfun  Parameters='BrakeUpd'  SFunctionDeploymentMode=off  EnableBusSupport=off
  BusCreator : BusCreator  Inputs=12
  CreateBus Vhcl.Wheel.PT : Subsystem
  Demux : Demux  Outputs=12
  Sync_Out : Outport
  Vhcl.Wheel.PT : Outport  Port=2
  wires:
  BrakeUpd/1 -> Sync_Out/1
  Brake/1 -> BrakeUpd/1  "Sync"
  Brake.IF.In/1 -> Brake/2
  VhclCtrl.Brake/1 -> Brake/3
  Brake/2 -> Demux/1
  BusCreator/1 -> BrakeUpd/2
  Sync_In/1 -> Brake/1
  Demux/12 -> BusCreator/12  "Brake IF Trq_Reg_trg RR"
  Demux/11 -> BusCreator/11  "Brake IF Trq_Reg_trg RL"
  Demux/10 -> BusCreator/10  "Brake IF Trq_Reg_trg FR"
  Demux/9 -> BusCreator/9  "Brake IF Trq_Reg_trg FL"
  Demux/8 -> BusCreator/8  "Brake IF Trq_PB RR"
  Demux/7 -> BusCreator/7  "Brake IF Trq_PB RL"
  Demux/6 -> BusCreator/6  "Brake IF Trq_PB FR"
  Demux/5 -> BusCreator/5  "Brake IF Trq_PB FL"
  Demux/4 -> BusCreator/4  "Brake IF Trq_WB RR"
  Demux/3 -> BusCreator/3  "Brake IF Trq_WB RL"
  Demux/2 -> BusCreator/2  "Brake IF Trq_WB FR"
  Demux/1 -> BusCreator/1  "Brake IF Trq_WB FL"
  BrakeUpd/2 -> CreateBus Vhcl.Wheel.PT/1(In)
  CreateBus Vhcl.Wheel.PT/1(Out) -> Vhcl.Wheel.PT/1

== system Torque_Vectoring_Controller_Boon/CarMaker/IPG Vehicle/CarAndTrailer ==
  Sync_In : Inport
  VhclCtrl.Steering : Inport  Port=2
  Vhcl.Wheel.In : Inport  Port=3
  Vhcl.Misc : Inport  Port=4
  CarAndTrailerUpd : Subsystem
  Forces : Subsystem
  Ground : Ground
  Kinematics : Subsystem
  Kinetics : Subsystem
  Steering : Subsystem
  Terminator : Terminator
  Terminator1 : Terminator
  Trailer : Subsystem
  Sync_Out : Outport
  Brake.IF.In : Outport  Port=2
  wires:
  Trailer/9(Car.Hitch.FrcTrq) -> CarAndTrailerUpd/9(Car.Hitch.FrcTrq)
  Trailer/8(Vhcl.Wheel.RR) -> CarAndTrailerUpd/8(Vhcl.Wheel.RR)
  Trailer/7(Vhcl.Wheel.RL) -> CarAndTrailerUpd/7(Vhcl.Wheel.RL)
  Trailer/6(Vhcl.Wheel.FR) -> CarAndTrailerUpd/6(Vhcl.Wheel.FR)
  Trailer/5(Vhcl.Wheel.FL) -> CarAndTrailerUpd/5(Vhcl.Wheel.FL)
  Trailer/4(Vhcl.PoI) -> CarAndTrailerUpd/4(Vhcl.PoI)
  Trailer/3(Vhcl.Motion) -> CarAndTrailerUpd/3(Vhcl.Motion)
  Trailer/2(Vhcl.Steering) -> CarAndTrailerUpd/2(Vhcl.Steering)
  Trailer/1(Sync_Out) -> CarAndTrailerUpd/1(Sync_In)
  CarAndTrailerUpd/2(Brake.IF.In) -> Brake.IF.In/1
  CarAndTrailerUpd/1(Sync_Out) -> Sync_Out/1
  Vhcl.Misc/1 -> Terminator1/1
  Vhcl.Wheel.In/1 -> Terminator/1
  Kinetics/6(WheelCarrier.Misc) -> Trailer/6(WheelCarrier.Misc)
  Kinetics/5(Car.Trq_T2W) -> Trailer/5(Car.Trq_T2W)
  Steering/2(Steer.IF) -> Kinematics/2(Steer.IF)
  Kinetics/4(Car.Fr1) -> Trailer/4(Car.Fr1)
  Kinetics/3(Car.Hitch) -> Trailer/3(Car.Hitch)
  Kinetics/2(Trailer.Load) -> Trailer/2(Trailer.Load)
  VhclCtrl.Steering/1 -> Steering/2(VhclCtrl.Steering)
  Sync_In/1 -> Steering/1(Sync_In)
  Steering/1(Sync_Out) -> Kinematics/1(Sync_In)
  Kinetics/1(Sync_Out) -> Trailer/1(Sync_In)
  Ground/1 -> CarAndTrailerUpd/10(Vhcl.Fr1A)
  Forces/11(FStabi) -> Kinetics/11(FStabi)
  Forces/10(FDamp) -> Kinetics/10(FDamp)
  Forces/9(FSpring) -> Kinetics/9(FSpring)
  Forces/8(TireRR_Out) -> Kinetics/8(TireRR.Out)
  Forces/7(TireRL_Out) -> Kinetics/7(TireRL.Out)
  Forces/6(TireFR_Out) -> Kinetics/6(TireFR.Out)
  Forces/5(TireFL_Out) -> Kinetics/5(TireFL.Out)
  Forces/4(Car.Load) -> Kinetics/4(Car.Load)
  Forces/2(Car.Virtual) -> Kinetics/2(Car.Virtual)
  Kinematics/6(lSpring) -> Forces/6(lSpring)
  Kinematics/7(vDamp) -> Forces/7(vDamp)
  Forces/3(Car.Aero) -> Kinetics/3(Car.Aero)
  Forces/1(Sync_Out) -> Kinetics/1(Sync_In)
  Kinematics/5(TireRR_In) -> Forces/5(TireRR_In)
  Kinematics/4(TireRL_In) -> Forces/4(TireRL_In)
  Kinematics/3(TireFR_In) -> Forces/3(TireFR_In)
  Kinematics/2(TireFL_In) -> Forces/2(TireFL_In)
  Kinematics/1(Sync_Out) -> Forces/1(Sync_In)
  Kinematics/8(lStabi) -> Forces/8(lStabi)
  Forces/12(FBuf) -> Kinetics/12(FBuf)
  Kinematics/9(lBuf) -> Forces/9(lBuf)

== system Torque_Vectoring_Controller_Boon/CarMaker/IPG Vehicle/PowerTrain ==
  note: When replacing the entire powertrain,
      | be sure to add '-disablepowertrain' to the command line arguments
      | in the CarMaker Model Configuration block.
  note: <Your model here>
  Sync_In : Inport
  Vhcl.Wheel.PT : Inport  Port=2
  VhclCtrl.PT : Inport  Port=3
  BusCreator1 : BusCreator  Inputs=40
  Constant : Constant  Value=4
  Constant1 : Constant  Value=0
  Demux1 : Demux  Outputs=40
  PowerTrain : S-Function  FunctionName=CM_Sfun  Parameters='PowerTrain'  SFunctionDeploymentMode=off  EnableBusSupport=off
  PowerTrainUpd : S-Function  FunctionName=CM_Sfun  Parameters='PowerTrainUpd'  SFunctionDeploymentMode=off  EnableBusSupport=off
  Terminator : Terminator
  Terminator1 : Terminator
  Sync_Out : Outport
  wires:
  Sync_In/1 -> PowerTrain/1
  PowerTrainUpd/1 -> Sync_Out/1
  VhclCtrl.PT/1 -> PowerTrain/3
  Vhcl.Wheel.PT/1 -> PowerTrain/2
  PowerTrain/2 -> Demux1/1
  BusCreator1/1 -> PowerTrainUpd/2
  Demux1/1 -> BusCreator1/1  "PT IF Ignition"
  Demux1/3 -> BusCreator1/3  "PT IF OperationError"
  Demux1/4 -> BusCreator1/4  "PT IF GearNo"
  Demux1/6 -> BusCreator1/6  "PT IF Engine_Trq (EngineControl)"
  Demux1/7 -> BusCreator1/7  "PT IF Trq_Supp2Bdy1 x"
  Demux1/8 -> BusCreator1/8  "PT IF Trq_Supp2Bdy1 y"
  Demux1/9 -> BusCreator1/9  "PT IF Trq_Supp2Bdy1 z"
  Demux1/10 -> BusCreator1/10  "PT IF Trq_Supp2BdyEng x"
  Demux1/11 -> BusCreator1/11  "PT IF Trq_Supp2BdyEng y"
  Demux1/12 -> BusCreator1/12  "PT IF DL_iDiff_mean"
  Demux1/13 -> BusCreator1/13  "PT IF WFL rot"
  Demux1/14 -> BusCreator1/14  "PT IF WFL rotv"
  Demux1/15 -> BusCreator1/15  "PT IF WFL Trq_B2W"
  Demux1/16 -> BusCreator1/16  "PT IF WFL Trq_Drive"
  Demux1/17 -> BusCreator1/17  "PT IF WFL Trq_Supp2WC"
  Demux1/18 -> BusCreator1/18  "PT IF WFL Trq_BrakeReg"
  Demux1/19 -> BusCreator1/19  "PT IF WFL Trq_BrakeReg_max"
  Demux1/20 -> BusCreator1/20  "PT IF WFR rot"
  Demux1/21 -> BusCreator1/21  "PT IF WFR rotv"
  Demux1/22 -> BusCreator1/22  "PT IF WFR Trq_B2W"
  Demux1/23 -> BusCreator1/23  "PT IF WFR Trq_Drive"
  Demux1/24 -> BusCreator1/24  "PT IF WFR Trq_Supp2WC"
  Demux1/25 -> BusCreator1/25  "PT IF WFR Trq_BrakeReg"
  Demux1/26 -> BusCreator1/26  "PT IF WFR Trq_BrakeReg_max"
  Demux1/27 -> BusCreator1/27  "PT IF WRL rot"
  Demux1/28 -> BusCreator1/28  "PT IF WRL rotv"
  Demux1/29 -> BusCreator1/29  "PT IF WRL Trq_B2W"
  Demux1/30 -> BusCreator1/30  "PT IF WRL Trq_Drive"
  Demux1/31 -> BusCreator1/31  "PT IF WRL Trq_Supp2WC"
  Demux1/32 -> BusCreator1/32  "PT IF WRL Trq_BrakeReg"
  Demux1/33 -> BusCreator1/33  "PT IF WRL Trq_BrakeReg_max"
  Demux1/34 -> BusCreator1/34  "PT IF WRR rot"
  Demux1/35 -> BusCreator1/35  "PT IF WRR rotv"
  Demux1/36 -> BusCreator1/36  "PT IF WRR Trq_B2W"
  Demux1/37 -> BusCreator1/37  "PT IF WRR Trq_Drive"
  Demux1/38 -> BusCreator1/38  "PT IF WRR Trq_Supp2WC"
  Demux1/39 -> BusCreator1/39  "PT IF WRR Trq_BrakeReg"
  Demux1/40 -> BusCreator1/40  "PT IF WRR Trq_BrakeReg_max"
  Demux1/2 -> Terminator/1  "PT IF OperationState"
  Constant/1 -> BusCreator1/2
  Demux1/5 -> Terminator1/1  "PT IF Engine_rotv"
  Constant1/1 -> BusCreator1/5
  PowerTrain/1 -> PowerTrainUpd/1  "Sync"

== system Torque_Vectoring_Controller_Boon/CarMaker/Vehicle Sensors/Subsystem ==
  "Sensors Scope " : Inport
  Bus Creator2 : BusCreator  Inputs=2
  Bus Selector : BusSelector  OutputSignals=ax,ay,wheelspeed,yawRate,wheelAngles,throttle,brake
  Bus Selector1 : BusSelector  OutputSignals=torque
  Scope : Scope
  Sensor Scope : Scope  NumInputPorts=6
  wires:
  Bus Selector/2 -> Bus Creator2/2  "<ay>"
  Bus Selector/4 -> Sensor Scope/3  "<yawRate>"
  Bus Selector/1 -> Bus Creator2/1  "<ax>"
  Bus Selector/6 -> Sensor Scope/5  "<throttle>"
  Bus Selector/7 -> Sensor Scope/6  "<brake>"
  Bus Selector/3 -> Sensor Scope/2  "<wheelspeed>"
  Bus Creator2/1 -> Sensor Scope/1
  "Sensors Scope "/1 -> Bus Selector1/1, Bus Selector/1
  Bus Selector/5 -> Sensor Scope/4  "<wheelAngles>"
  Bus Selector1/1 -> Scope/1  "<torque>"

== system Torque_Vectoring_Controller_Boon/CarMaker/VehicleControl/CreateBus Vhcl.Misc ==
  In1 : Inport
  Bus Creator5 : BusCreator  Inputs=11
  Demux5 : Demux  Outputs=11
  Out1 : Outport
  wires:
  Demux5/11 -> Bus Creator5/11  "Vhcl Wind_vel_0 z"
  Demux5/10 -> Bus Creator5/10  "Vhcl Wind_vel_0 y"
  Demux5/9 -> Bus Creator5/9  "Vhcl Wind_vel_0 x"
  Demux5/8 -> Bus Creator5/8  "Vhcl DL2BdyEng y"
  Demux5/7 -> Bus Creator5/7  "Vhcl DL2BdyEng x"
  Demux5/6 -> Bus Creator5/6  "Vhcl TrqDL2Bdy1B z"
  Demux5/5 -> Bus Creator5/5  "Vhcl TrqDL2Bdy1B y"
  Demux5/4 -> Bus Creator5/4  "Vhcl TrqDL2Bdy1B x"
  Demux5/3 -> Bus Creator5/3  "Vhcl Trq_DL2Bdy1 z"
  In1/1 -> Demux5/1
  Bus Creator5/1 -> Out1/1
  Demux5/2 -> Bus Creator5/2  "Vhcl Trq_DL2Bdy1 y"
  Demux5/1 -> Bus Creator5/1  "Vhcl Trq_DL2Bdy1 x"

== system Torque_Vectoring_Controller_Boon/CarMaker/VehicleControl/CreateBus Vhcl.Wheel.In ==
  In1 : Inport
  Bus Creator1 : BusCreator  Inputs=12
  Demux1 : Demux  Outputs=12
  Out1 : Outport
  wires:
  Demux1/12 -> Bus Creator1/12  "Vhcl Wheel RR rotv"
  Demux1/11 -> Bus Creator1/11  "Vhcl Wheel RR Trq_DL2WC"
  Demux1/10 -> Bus Creator1/10  "Vhcl Wheel RR Trq_B2WC"
  Demux1/9 -> Bus Creator1/9  "Vhcl Wheel RL rotv"
  Demux1/8 -> Bus Creator1/8  "Vhcl Wheel RL Trq_DL2WC"
  Demux1/7 -> Bus Creator1/7  "Vhcl Wheel RL Trq_B2WC"
  Demux1/6 -> Bus Creator1/6  "Vhcl Wheel FR rotv"
  Demux1/5 -> Bus Creator1/5  "Vhcl Wheel FR Trq_DL2WC"
  Demux1/4 -> Bus Creator1/4  "Vhcl Wheel FR Trq_B2WC"
  Demux1/3 -> Bus Creator1/3  "Vhcl Wheel FL rotv"
  In1/1 -> Demux1/1
  Bus Creator1/1 -> Out1/1
  Demux1/2 -> Bus Creator1/2  "Vhcl Wheel FL Trq_DL2WC"
  Demux1/1 -> Bus Creator1/1  "Vhcl Wheel FL Trq_B2WC"

== system Torque_Vectoring_Controller_Boon/CarMaker/VehicleControl/CreateBus VhclCtrl ==
  In : Inport
  BusCreator : BusCreator  Inputs=29
  Demux : Demux  Outputs=29
  Out : Outport
  wires:
  In/1 -> Demux/1
  BusCreator/1 -> Out/1
  Demux/1 -> BusCreator/1  "VhclCtrl SST"
  Demux/2 -> BusCreator/2  "VhclCtrl Key"
  Demux/3 -> BusCreator/3  "VhclCtrl UserSignal0"
  Demux/4 -> BusCreator/4  "VhclCtrl UserSignal1"
  Demux/5 -> BusCreator/5  "VhclCtrl UserSignal2"
  Demux/6 -> BusCreator/6  "VhclCtrl UserSignal3"
  Demux/7 -> BusCreator/7  "VhclCtrl UserSignal4"
  Demux/8 -> BusCreator/8  "VhclCtrl GearNo"
  Demux/9 -> BusCreator/9  "VhclCtrl SelectorCtrl"
  Demux/10 -> BusCreator/10  "VhclCtrl Brake"
  Demux/11 -> BusCreator/11  "VhclCtrl BrakePark"
  Demux/12 -> BusCreator/12  "VhclCtrl Clutch"
  Demux/13 -> BusCreator/13  "VhclCtrl Gas"
  Demux/14 -> BusCreator/14  "VhclCtrl Steering Ang"
  Demux/15 -> BusCreator/15  "VhclCtrl Steering AngVel"
  Demux/16 -> BusCreator/16  "VhclCtrl Steering AngAcc"
  Demux/17 -> BusCreator/17  "VhclCtrl Steering Trq"
  Demux/18 -> BusCreator/18  "VhclCtrl Lights LowBeam"
  Demux/19 -> BusCreator/19  "VhclCtrl Lights HighBeam"
  Demux/20 -> BusCreator/20  "VhclCtrl Lights Daytime"
  Demux/21 -> BusCreator/21  "VhclCtrl Lights ParkL"
  Demux/22 -> BusCreator/22  "VhclCtrl Lights ParkR"
  Demux/23 -> BusCreator/23  "VhclCtrl Lights IndL"
  Demux/24 -> BusCreator/24  "VhclCtrl Lights IndR"
  Demux/25 -> BusCreator/25  "VhclCtrl Lights FogFrontL"
  Demux/26 -> BusCreator/26  "VhclCtrl Lights FogFrontR"
  Demux/27 -> BusCreator/27  "VhclCtrl Lights FogRear"
  Demux/28 -> BusCreator/28  "VhclCtrl Lights Brake"
  Demux/29 -> BusCreator/29  "VhclCtrl Lights Reverse"

== system Torque_Vectoring_Controller_Boon/CarMaker/VehicleControl/CreateBus VhclCtrl.PT ==
  In1 : Inport
  BusCreator : BusCreator  Inputs=11
  Demux : Demux  Outputs=11
  Out1 : Outport
  wires:
  In1/1 -> Demux/1
  BusCreator/1 -> Out1/1
  Demux/1 -> BusCreator/1  "VhclCtrl SST"
  Demux/2 -> BusCreator/2  "VhclCtrl Key"
  Demux/3 -> BusCreator/3  "VhclCtrl UserSignal0"
  Demux/4 -> BusCreator/4  "VhclCtrl UserSignal1"
  Demux/5 -> BusCreator/5  "VhclCtrl UserSignal2"
  Demux/6 -> BusCreator/6  "VhclCtrl UserSignal3"
  Demux/7 -> BusCreator/7  "VhclCtrl UserSignal4"
  Demux/8 -> BusCreator/8  "VhclCtrl GearNo"
  Demux/9 -> BusCreator/9  "VhclCtrl SelectorCtrl"
  Demux/10 -> BusCreator/10  "VhclCtrl Clutch"
  Demux/11 -> BusCreator/11  "VhclCtrl Gas"

== system Torque_Vectoring_Controller_Boon/CarMaker/VehicleControl/CreateBus VhclCtrl.Steering ==
  In1 : Inport
  Bus Creator : BusCreator  Inputs=5
  Demux : Demux  Outputs=5
  Out1 : Outport
  wires:
  In1/1 -> Demux/1
  Bus Creator/1 -> Out1/1
  Demux/1 -> Bus Creator/1  "VhclCtrl Steering Ang"
  Demux/5 -> Bus Creator/5  "VhclCtrl Steering ByTrq"
  Demux/3 -> Bus Creator/3  "VhclCtrl Steering AngAcc"
  Demux/2 -> Bus Creator/2  "VhclCtrl Steering AngVel"
  Demux/4 -> Bus Creator/4  "VhclCtrl Steering Trq"

== system Torque_Vectoring_Controller_Boon/CarMaker/Controls/Control Systems/Distributor ==
  sensors : Inport
  settings : Inport  Port=2
  estimPar : Inport  Port=3
  variables : Inport  Port=4
  Mz : Inport  Port=5
  MATLAB Function : MATLAB Function  TreatAsAtomicUnit=on
  MdesFdesFxmaxFx : Scope  NumInputPorts=4
  Mux : Mux
  To Workspace : ToWorkspace  VariableName=Fdes  SaveFormat=Timeseries  SampleTime=-1
  To Workspace1 : ToWorkspace  VariableName=Fxmax  SaveFormat=Timeseries  SampleTime=-1
  To Workspace2 : ToWorkspace  VariableName=MdesFdesFxmaxFx  SaveFormat=Timeseries  SampleTime=-1
  To Workspace4 : ToWorkspace  VariableName=Fx  SaveFormat=Timeseries  SampleTime=-1
  torqueDistribution : Outport
  slipSet : Outport  Port=2
  wires:
  MATLAB Function/1(torqueDistribution) -> torqueDistribution/1
  sensors/1 -> MATLAB Function/1(sensors)
  settings/1 -> MATLAB Function/2(settings)
  estimPar/1 -> MATLAB Function/3(estimPar)
  Mz/1 -> Mux/1, MATLAB Function/5(Mz)
  MATLAB Function/2(slipSet) -> slipSet/1
  variables/1 -> MATLAB Function/4(variables)
  MATLAB Function/3(Fdes) -> Mux/2, MdesFdesFxmaxFx/1, To Workspace/1
  MATLAB Function/4(sumFx) -> MdesFdesFxmaxFx/2
  MATLAB Function/6(Fxmaxsum) -> MdesFdesFxmaxFx/4
  Mux/1 -> To Workspace2/1
  MATLAB Function/7(Fx) -> To Workspace4/1, Mux/4
  MATLAB Function/5(Fxmax) -> To Workspace1/1, MdesFdesFxmaxFx/3, Mux/3

== system Torque_Vectoring_Controller_Boon/CarMaker/Controls/Control Systems/Traction Controller ==
  Sensor Bus : Inport
  Estim Par Bus : Inport  Port=2
  Max Traction Force : Subsystem
  slip ratio : Subsystem
  Out1 : Outport
  wires:
  Max Traction Force/1(" Max Traction Force Bus") -> ?
  Estim Par Bus/1 -> Max Traction Force/1(Estim Par Bus)
  Sensor Bus/1 -> slip ratio/1(sensor bus)
  ? -> ?

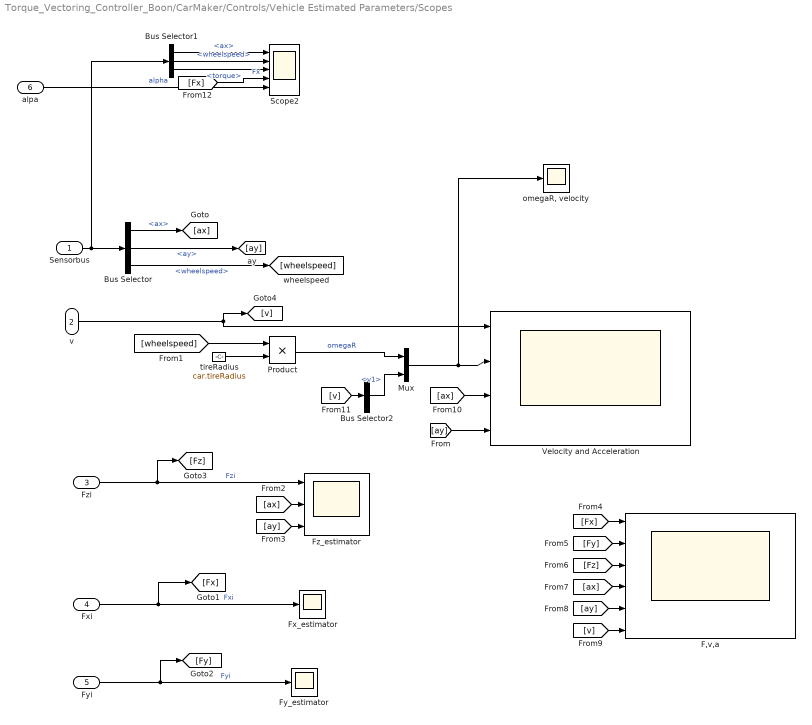
== system Torque_Vectoring_Controller_Boon/CarMaker/Controls/Vehicle Estimated Parameters/Scopes ==
  Sensorbus : Inport
  v : Inport  Port=2
  Fzi : Inport  Port=3
  Fxi : Inport  Port=4
  Fyi : Inport  Port=5
  alpa : Inport  Port=6
  Bus Selector : BusSelector  OutputSignals=ax,ay,wheelspeed
  Bus Selector1 : BusSelector  OutputSignals=ax,wheelspeed,torque
  Bus Selector2 : BusSelector  OutputSignals=v1
  F,v,a : Scope  NumInputPorts=6
  Fx_estimator : Scope
  Fy_estimator : Scope
  Fz_estimator : Scope  NumInputPorts=3
  Mux : Mux  Inputs=2
  Product : Product
  Scope2 : Scope  NumInputPorts=5
  "Velocity and Acceleration " : Scope  NumInputPorts=4
  "omegaR, velocity" : Scope
  tireRadius : Constant  Value=car.tireRadius
  wires:
  tireRadius/1 -> Product/2
  Product/1 -> Mux/1  "omegaR"
  v/1 -> "Velocity and Acceleration "/1, [v]
  Fzi/1 -> [Fz], Fz_estimator/1  "Fzi"
  Sensorbus/1 -> Bus Selector1/1, Bus Selector/1
  Bus Selector/2 -> [ay]  "<ay>"
  [ay] -> "Velocity and Acceleration "/4
  Bus Selector/3 -> [wheelspeed]  "<wheelspeed>"
  [wheelspeed] -> Product/1
  Bus Selector/1 -> [ax]  "<ax>"
  [ax] -> Fz_estimator/2
  [ay] -> Fz_estimator/3
  Fxi/1 -> [Fx], Fx_estimator/1  "Fxi"
  Fyi/1 -> [Fy], Fy_estimator/1  "Fyi"
  [Fz] -> F,v,a/3
  [Fy] -> F,v,a/2
  [Fx] -> F,v,a/1
  [ax] -> F,v,a/4
  [ay] -> F,v,a/5
  [v] -> F,v,a/6
  [ax] -> "Velocity and Acceleration "/3
  [v] -> Bus Selector2/1
  Bus Selector2/1 -> Mux/2  "<v1>"
  Mux/1 -> "Velocity and Acceleration "/2, "omegaR, velocity"/1
  Bus Selector1/1 -> Scope2/1  "<ax>"
  Bus Selector1/2 -> Scope2/2  "<wheelspeed>"
  Bus Selector1/3 -> Scope2/3  "<torque>"
  [Fx] -> Scope2/4  "Fx"
  alpa/1 -> Scope2/5  "alpha"

== system Torque_Vectoring_Controller_Boon/CarMaker/Controls/Vehicle Estimated Parameters/Velocity Estimator ==
  Sensors : Inport
  Settings : Inport  Port=2
  Fyi : Inport  Port=3
  Bus Creator : BusCreator  Inputs=4
  Fuzzy Velocity : Subsystem
  Kalman Velocity : MATLAB Function  TreatAsAtomicUnit=on
  MATLAB Function : MATLAB Function  TreatAsAtomicUnit=on
  Memory : Memory
  Scope : Scope  NumInputPorts=3
  Signal Specification : SignalSpecification  Dimensions=[4,1]
  Sum : Sum  Inputs=+-
  Terminator2 : Terminator
  Velicity Estimator 2 : MATLAB Function  TreatAsAtomicUnit=on
  Velocity Estimator 1 : MATLAB Function  TreatAsAtomicUnit=on
  Velocity_Estimator3 : MATLAB Function  TreatAsAtomicUnit=on
  Velocity_Estimator4 : MATLAB Function  TreatAsAtomicUnit=on
  error : Scope
  v : Outport
  vBus : Outport  Port=2
  wires:
  Velocity Estimator 1/1(v1) -> Sum/1, MATLAB Function/1(v1), Bus Creator/1  "v1"
  Sensors/1 -> Fuzzy Velocity/1(Sensors), Kalman Velocity/1(sensors), Velocity_Estimator4/1(sensors), Velocity_Estimator3/1(sensors), Velicity Estimator 2/1(sensors), Velocity Estimator 1/1(sensors)  "sensors"
  Settings/1 -> Fuzzy Velocity/2(Settings), Kalman Velocity/2(settings), Velocity_Estimator4/2(settings), Velocity_Estimator3/2(settings), Velicity Estimator 2/2(settings), Velocity Estimator 1/2(settings)  "settings"
  Velocity_Estimator3/1(v3) -> Bus Creator/3, MATLAB Function/3(v3), Sum/2  "v3"
  Bus Creator/1 -> vBus/1  "vBus"
  Velicity Estimator 2/1(v2) -> Kalman Velocity/3(v2), Scope/1, MATLAB Function/2(v2), Bus Creator/2
  MATLAB Function/1(v) -> Memory/1, v/1
  Memory/1 -> Velocity_Estimator3/3(v)
  Sum/1 -> error/1
  Velicity Estimator 2/2(vCOG) -> Terminator2/1
  Fyi/1 -> Signal Specification/1
  Velocity_Estimator4/1(v4) -> Kalman Velocity/4(v4), Bus Creator/4, MATLAB Function/4(v4), Scope/2
  Signal Specification/1 -> Velocity_Estimator4/3(Fyi)
  Kalman Velocity/1(vKalman) -> MATLAB Function/5(vKalman), Scope/3
  Fuzzy Velocity/1(vFuzzy) -> MATLAB Function/6(vFuzzy)

== system Torque_Vectoring_Controller_Boon/CarMaker/IPG Feedback/Subsystem/CreateBus PTC ClutchOut ==
  In : Inport
  BusCreator : BusCreator  Inputs=3
  Demux : Demux  Outputs=3
  Out : Outport
  wires:
  In/1 -> Demux/1
  BusCreator/1 -> Out/1
  Demux/1 -> BusCreator/1  "PTC ClutchOut Pos"
  Demux/2 -> BusCreator/2  "PTC ClutchOut rotv_out_trg"
  Demux/3 -> BusCreator/3  "PTC ClutchOut Trq_out_trg"
